simulink model "dspqdemo"  (Simulink 8.3)
settings: Solver=FixedStepDiscrete  StartTime=0.0  StopTime=inf  RelTol=1e-3
libraries: dspmisc x1, dspbuff3 x1, dspsigops x1
settings Model: Creator=The MathWorks Inc.  ExtModeTrigMode=oneshot  ExtModeArmWhenConnect=off
settings DataIOCC: LimitDataPoints=off  SaveOutput=off  SaveTime=off
settings OptimizationCC: BlockReduction=off  BooleanDataType=off  ExpressionDepthLimit=2147483647  InitFltsAndDblsToZero=on  BufferReusableBoundary=off
settings DebuggingCC: SignalResolutionControl=TryResolveAllWithWarning  SolverPrmCheckMsg=none  MultiTaskDSMMsg=warning  MultiTaskCondExecSysMsg=none  IntegerOverflowMsg=none  FcnCallInpInsideContextMsg=UseLocalSettings  BusObjectLabelMismatch=none  StrictBusMsg=None
settings HardwareCC: TargetUnknown=on
settings RTWCC: RetainRTWFile=on  IncludeERTFirstTime=on

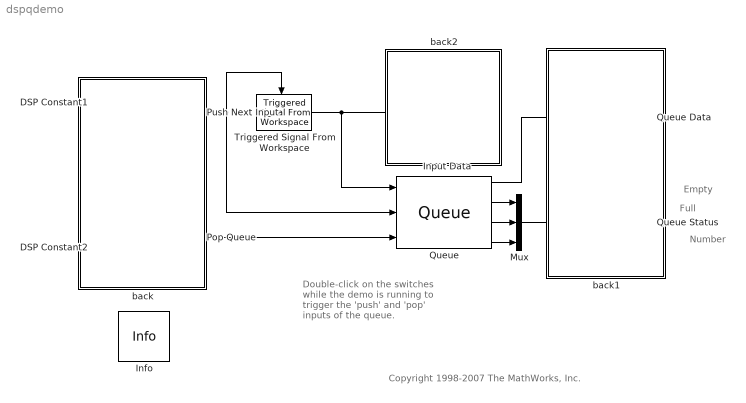
== system dspqdemo ==
  note: Number
  note: Full
  note: Empty
  note: Double-click on the switches
      | while the demo is running
      | to trigger the 'push' and 'pop'
      | inputs of the queue.
  note: Copyright 1998-2007 The MathWorks, Inc.
  DSP Constant1 : Constant  SampleTime=4
  DSP Constant2 : Constant  Value=0  SampleTime=4
  Info : dspmisc/Info  SystemSampleTime=-1
  Input Data : Display
  Mux : Mux  Inputs=3
  Pop Queue : ManualSwitch
  Push Next Input : ManualSwitch
  Queue : dspbuff3/Queue  depth=3  trigger=Either edge  overflow=Warning  pes=Warning  eso=on  fso=on  nso=on  clr=off  clrOutport=on  adf=on
  Queue Data : Display
  Queue Status : Display
  Triggered Signal From Workspace : dspsigops/Triggered Signal From Workspace  Signal=1:32  TriggerType=Either edge  ic=0  SamplesPerFrame=4  OutputAfterFinalValue=Setting to zero
  back : Subsystem
  back1 : Subsystem
  back2 : Subsystem
  wires:
  Pop Queue/1 -> Queue/3
  Queue/3 -> Mux/2
  Queue/2 -> Mux/1
  Queue/4 -> Mux/3
  Mux/1 -> Queue Status/1
  Push Next Input/1 -> Queue/2, Triggered Signal From Workspace/Trigger
  DSP Constant1/1 -> Pop Queue/1, Push Next Input/1
  DSP Constant2/1 -> Pop Queue/2, Push Next Input/2
  Queue/1 -> Queue Data/1
  Triggered Signal From Workspace/1 -> Input Data/1, Queue/1

== system dspqdemo/back ==

== system dspqdemo/back1 ==

== system dspqdemo/back2 ==
